simulink model "DIGITAL_TWIN_MPC"  (R2023b)
settings: Solver=FixedStepAuto  StartTime=0.0  StopTime=inf  FixedStep=0.005  RelTol=1e-3  EnableMultiTasking=on
undefined symbols (not defined in the file or in its folder): DiscIntNeverNeededParam, HIL, qc_get_step_size
libraries: quarc_library x6
settings Model: ExtModeTrigDuration=10000  Creator=franc  LastModifiedBy=franc
settings SolverCC: AlgebraicLoopSolver=TrustRegion  PositivePriorityOrder=on
settings DataIOCC: ReturnWorkspaceOutputs=off
settings OptimizationCC: LifeSpan=inf
settings DebuggingCC: UnconnectedInputMsg=warning  UnconnectedOutputMsg=warning  UnconnectedLineMsg=warning  ArithmeticOperatorsInVariantConditions=warning
settings ModelReferenceCC: EnableRefExpFcnMdlSchedulingChecks=on
settings SFSimCC: SimUseLocalCustomCode=off  CustomCodeUndefinedFunction=UseInterfaceOnly
settings RTWCC: Description=QUARC Win64 Target  SystemTargetFile=quarc_win64.tlc  TemplateMakefile=quarc_default_tmf  RTWUseLocalCustomCode=off
settings CodeAppCC: StateflowObjectComments=on
settings STFCustomTargetCC: TargetPreCompLibLocation=C:\PROGRA~3\QUARC\lib\2016a\win64\release  ConcurrentExecutionCompliant=on  GRTInterface=on  SystemTargetFile=quarc_win64.tlc
settings GRTTargetCC: TargetPreCompLibLocation=C:\PROGRA~3\QUARC\lib\2016a\win64\release  ParMdlRefBuildCompliant=off  CompOptLevelCompliant=off  CombineOutputUpdateFcns=off  MatFileLogging=off  CPPClassGenCompliant=off  GRTInterface=on  UseToolchainInfoCompliant=off  ExtMode=on  ExtModeMexFile=quarc_comm
settings ConfigComp: CovMetricSettings=dswe

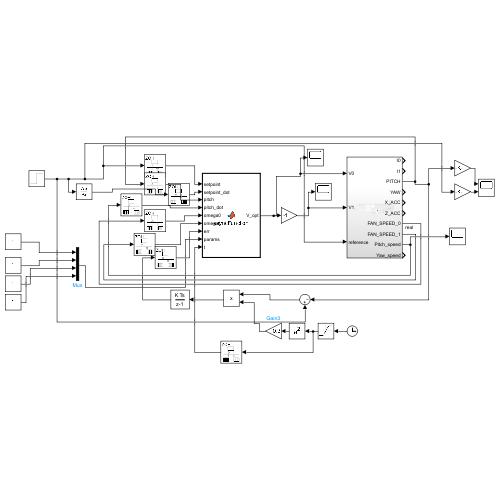
[thumbnail: Simulink's stored preview of the top-level diagram]
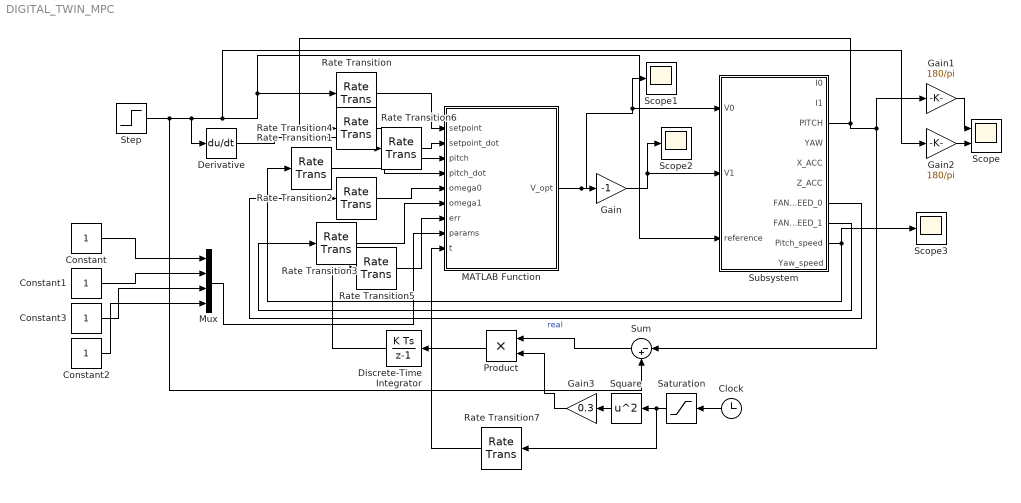
== system DIGITAL_TWIN_MPC ==
  Clock : Clock
  Constant{,1..3} (4 alike) : Constant
  Derivative : Derivative
  Discrete-Time Integrator : DiscreteIntegrator  SampleTime=-1  ICPrevOutput=DiscIntNeverNeededParam  ICPrevScaledInput=DiscIntNeverNeededParam
  Gain : Gain  Gain=-1
  Gain1 : Gain  Gain=180/pi
  Gain2 : Gain  Gain=180/pi
  Gain3 : Gain  Gain=0.3
  MATLAB Function : MATLAB Function  TreatAsAtomicUnit=on  SystemSampleTime=0.1
  Mux : Mux
  Product : Product
  Rate Transition{,1..7} (8 alike) : RateTransition
  Saturation : Saturate  UpperLimit=10  LowerLimit=0
  Scope : Scope  NumInputPorts=2
  Scope1 : Scope
  Scope2 : Scope
  Scope3 : Scope
  Square : Math  Operator=square
  Step : Step  After=30*pi/180  SampleTime=0
  Subsystem : Subsystem
  Sum : Sum  Inputs=|-+
  wires:
  Derivative/1 -> Rate Transition6/1
  Rate Transition4/1 -> MATLAB Function/3(pitch)
  Subsystem/9(Pitch_speed) -> Rate Transition1/1, Scope3/1
  Subsystem/7(FAN_SPEED_0) -> Rate Transition2/1  "real"
  Step/1 -> Sum/2, Derivative/1, Gain2/1, Subsystem/3(reference), Rate Transition/1
  Rate Transition5/1 -> MATLAB Function/7(err)
  Sum/1 -> Product/1
  Discrete-Time Integrator/1 -> Rate Transition5/1
  Gain/1 -> Subsystem/2(V1), Scope2/1
  Rate Transition1/1 -> MATLAB Function/4(pitch_dot)
  Subsystem/8(FAN_SPEED_1) -> Rate Transition3/1
  Rate Transition2/1 -> MATLAB Function/5(omega0)
  MATLAB Function/1(V_opt) -> Gain/1, Scope1/1, Subsystem/1(V0)
  Rate Transition/1 -> MATLAB Function/1(setpoint)
  Rate Transition3/1 -> MATLAB Function/6(omega1)
  Rate Transition6/1 -> MATLAB Function/2(setpoint_dot)
  Subsystem/3(PITCH) -> Gain1/1, Sum/1, Rate Transition4/1
  Gain1/1 -> Scope/1
  Gain2/1 -> Scope/2
  Mux/1 -> MATLAB Function/8(params)
  Rate Transition7/1 -> MATLAB Function/9(t)
  Constant/1 -> Mux/1
  Constant1/1 -> Mux/2
  Constant3/1 -> Mux/3
  Constant2/1 -> Mux/4
  Product/1 -> Discrete-Time Integrator/1
  Saturation/1 -> Rate Transition7/1, Square/1
  Square/1 -> Gain3/1
  Gain3/1 -> Product/2
  Clock/1 -> Saturation/1

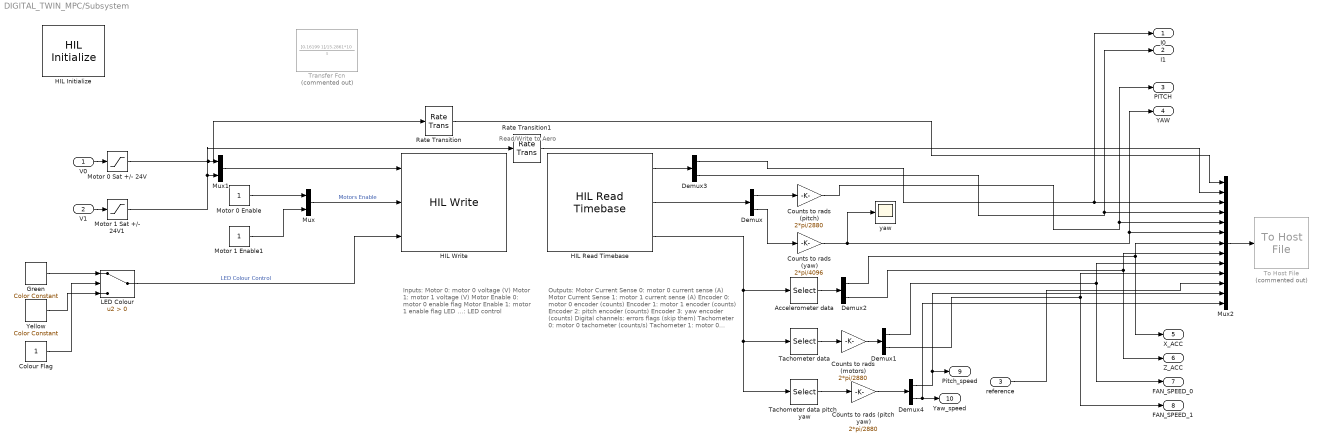
== system DIGITAL_TWIN_MPC/Subsystem ==
  note: Read/Write to Aero
  note: Outputs:
      | Motor Current Sense 0: motor 0 current sense (A)
      | Motor Current Sense 1: motor 1 current sense (A)
      |
      | Encoder 0: motor 0 encoder (counts)
      | Encoder 1: motor 1 encoder (counts)
      | Encoder 2: pitch encoder (counts)
      | Encoder 3: yaw encoder (counts)
      |
      | Digital channels: errors flags (skip them)
      |
      | Tachometer 0: motor 0 tachometer (counts/s)
      | Tachometer 1: motor 0 tachometer (counts/s)
      | Tachometer 2: pitch tachometer (counts/s)
      | Tachometer 3: yaw tachometer (counts/s)
      | Gyro X axis: angular velocity about X axis (rad/s)
      | Gyro Y axis: angular velocity about Y axis (rad/s)
      | Gyro Z axis: angular velocity about Z axis (rad/s)
      | Acceleration X axis: acceleration along X axis (m/s^2)
      | Acceleration Y axis: acceleration along Y axis (m/s^2)
      | Acceleration Z axis: acceleration along Z axis (m/s^2)
  note: Inputs:
      | 	Motor 0: motor 0 voltage (V)
      | 	Motor 1: motor 1 voltage (V)
      |
      | 	Motor Enable 0: motor 0 enable flag
      | 	Motor Enable 1: motor 1 enable flag
      |
      | 	LED ...: LED control
  V0 : Inport
  V1 : Inport  Port=2
  reference : Inport  Port=3
  Accelerometer data : Selector  InputPortWidth=6  IndexOptions=Index vector (dialog)  Indices=[1 2]  OutputSizes=1
  Colour Flag : Constant
  Counts to rads (motors) : Gain  Gain=2*pi/2880
  Counts to rads (pitch yaw) : Gain  Gain=2*pi/2880
  Counts to rads (pitch) : Gain  Gain=2*pi/2880
  Counts to rads (yaw) : Gain  Gain=2*pi/4096
  Demux{,1..4} (5 alike) : Demux  Outputs=2
  Green : quarc_library/Sources/Signals/Color Constant  color=[0 1 0]
      settings: SourceProductName=QUARC Targets
  HIL Initialize : quarc_library/Data Acquisition/Generic/Configuration/HIL Initialize  Priority=-99  object_name=HIL-1  board_type=quanser_aero2_usb  board_number=0@tcpip://localhost:18950  board_options=""  exclusive=off  active=on  hardware_clocks=[0]  clock_modes=[]  initial_clock_frequencies=[]  set_clock_params_at_start=off  set_clock_params_at_switch_in=off  set_clock_frequencies_at_start=off  set_clock_frequencies_at_switch_in=off  analog_input_channels=[0:1]  analog_input_configurations=[]  analog_input_maximums=3  analog_input_minimums=-3  set_analog_input_params_at_start=off  set_analog_input_params_at_switch_in=off  analog_output_channels=[0:1]  analog_output_maximums=24  analog_output_minimums=-24  initial_analog_outputs=[0]  final_analog_outputs=[0]  watchdog_analog_outputs=[0]  set_analog_output_params_at_start=off  set_analog_output_params_at_switch_in=off  set_analog_outputs_at_start=on  set_analog_outputs_at_switch_in=off  set_analog_outputs_at_terminate=on  set_analog_outputs_at_switch_out=off  set_analog_outputs_on_watchdog=on  digital_input_channels=[]  digital_output_channels=[0:1]  digital_output_configuration=[]  initial_digital_outputs=[1]  final_digital_outputs=[0]  watchdog_digital_outputs=[0]  set_digital_output_params_at_start=off  set_digital_output_params_at_switch_in=off  set_digital_outputs_at_start=on  set_digital_outputs_at_switch_in=off  set_digital_outputs_at_terminate=on  set_digital_outputs_at_switch_out=off  set_digital_outputs_on_watchdog=on  encoder_channels=[0:3]  quadrature=[4]  encoder_filter_frequency=[]  initial_encoder_counts=[0]  set_encoder_params_at_start=off  set_encoder_params_at_switch_in=off  set_encoder_counts_at_start=on  set_encoder_counts_at_switch_in=off  pwm_channels=[]  pwm_modes=[]  pwm_frequency=[]  pwm_configuration=[]  pwm_alignment=[]  pwm_polarity=[]  pwm_leading_deadband=[]  pwm_trailing_deadband=[]  initial_pwm_outputs=[]  final_pwm_outputs=[]  watchdog_pwm_outputs=[]  set_pwm_params_at_start=off  set_pwm_params_at_switch_in=off  set_pwm_outputs_at_start=off  set_pwm_outputs_at_switch_in=off  set_pwm_outputs_at_terminate=off  set_pwm_outputs_at_switch_out=off  set_pwm_outputs_on_watchdog=off  other_output_channels=[11000:11002]  initial_other_outputs=[0 1 0]  final_other_outputs=[1 0 0]  watchdog_other_outputs=[0 0 1]  set_other_outputs_at_start=on  set_other_outputs_at_switch_in=off  set_other_outputs_at_terminate=on  set_other_outputs_at_switch_out=off  set_other_outputs_on_watchdog=on
  HIL Read Timebase : quarc_library/Data Acquisition/Generic/Timebases/HIL Read Timebase  object_name=HIL-1  clock=0  analog_channels=[0:1]  encoder_channels=[2:3]  digital_channels=[]  other_channels=[4000 4002 14000:14003 ]  active=on  vector_output=on  data_type_mode=Inherit via back propagation  encoder_data_type=double  digital_data_type=boolean  overflow_mode=Overwrite on overflow  samples_in_buffer=max(ceil(1/qc_get_step_size), 1)
  HIL Write : quarc_library/Data Acquisition/Generic/Immediate I//O/HIL Write  object_name=HIL-1  analog_channels=[0:1]  pwm_channels=[]  digital_channels=[0:1]  other_channels=[11000:11002]  sample_time=-1  active=on  vector_input=on
  LED Colour : Switch  Criteria=u2 > Threshold  SaturateOnIntegerOverflow=off  InputSameDT=off
  Motor 0 Enable : Constant
  Motor 0 Sat +/- 24V : Saturate  UpperLimit=18  LowerLimit=-18
  Motor 1 Enable1 : Constant
  Motor 1 Sat +/- 24V1 : Saturate  UpperLimit=18  LowerLimit=-18
  Mux : Mux  Inputs=2
  Mux1 : Mux  Inputs=2
  Mux2 : Mux  Inputs=13
  Rate Transition : RateTransition
  Rate Transition1 : RateTransition
  Tachometer data : Selector  InputPortWidth=6  IndexOptions=Index vector (dialog)  Indices=[3 4]  OutputSizes=1
  Tachometer data pitch_yaw : Selector  InputPortWidth=6  IndexOptions=Index vector (dialog)  Indices=[5 6]  OutputSizes=1
  To Host File : quarc_library/Sinks/To Host/To Host File  Commented=on  source=Specify via dialog (do not evaluate)  file_name=CONTROLLED_STEP.mat  variable_name=data  decimation=1  sample_time=-1  file_format=MAT-file v.4  options=No header or footer  append=off  final_file_name=CONTROLLED_STEP.mat  bitrate=2000000
  Transfer Fcn : TransferFcn  Commented=on  Numerator=[0.16199 1]/15.2861*10  Denominator=[1 0]
  Yellow : quarc_library/Sources/Signals/Color Constant  color=[1 1 0]
      settings: SourceProductName=QUARC Targets
  yaw : Scope
  I0 : Outport
  I1 : Outport  Port=2
  PITCH : Outport  Port=3
  YAW : Outport  Port=4
  X_ACC : Outport  Port=5
  Z_ACC : Outport  Port=6
  FAN_SPEED_0 : Outport  Port=7
  FAN_SPEED_1 : Outport  Port=8
  Pitch_speed : Outport  Port=9
  Yaw_speed : Outport  Port=10
  wires:
  Demux2/1 -> X_ACC/1, Mux2/7
  Demux2/2 -> Z_ACC/1, Mux2/8
  Demux1/2 -> FAN_SPEED_1/1, Mux2/10
  Demux/1 -> Counts to rads (pitch)/1
  Counts to rads (pitch)/1 -> PITCH/1, Mux2/5
  Motor 0 Sat +/- 24V/1 -> Mux1/1, Rate Transition/1
  Counts to rads (yaw)/1 -> YAW/1, Mux2/6, yaw/1
  Demux1/1 -> FAN_SPEED_0/1, Mux2/9
  Demux3/2 -> I1/1, Mux2/4
  LED Colour/1 -> HIL Write/3  "LED Colour Control"
  V1/1 -> Motor 1 Sat +/- 24V1/1
  HIL Read Timebase/3 -> Tachometer data pitch_yaw/1, Tachometer data/1, Accelerometer data/1
  Mux2/1 -> To Host File/1
  Demux3/1 -> I0/1, Mux2/3
  Counts to rads (motors)/1 -> Demux1/1
  Yellow/1 -> LED Colour/3
  Green/1 -> LED Colour/1
  Mux/1 -> HIL Write/2  "Motors Enable"
  Motor 1 Sat +/- 24V1/1 -> Mux1/2, Rate Transition1/1
  Motor 1 Enable1/1 -> Mux/2
  HIL Read Timebase/2 -> Demux/1
  HIL Read Timebase/1 -> Demux3/1
  Tachometer data/1 -> Counts to rads (motors)/1
  V0/1 -> Motor 0 Sat +/- 24V/1
  Mux1/1 -> HIL Write/1
  Colour Flag/1 -> LED Colour/2
  Demux/2 -> Counts to rads (yaw)/1
  Motor 0 Enable/1 -> Mux/1
  Accelerometer data/1 -> Demux2/1
  reference/1 -> Mux2/11
  Tachometer data pitch_yaw/1 -> Counts to rads (pitch yaw)/1
  Counts to rads (pitch yaw)/1 -> Demux4/1
  Demux4/1 -> Pitch_speed/1, Mux2/12
  Demux4/2 -> Yaw_speed/1, Mux2/13
  Rate Transition/1 -> Mux2/1
  Rate Transition1/1 -> Mux2/2

== matlab function DIGITAL_TWIN_MPC/MATLAB Function ==
  data: setpoint input; setpoint_dot input; V_opt output; pitch input; pitch_dot input; omega0 input; omega1 input; err input; params input; t input
function V_opt = asyncFunction(setpoint,setpoint_dot,pitch,pitch_dot,omega0,omega1,err,params,t)
    fun=@(V)simulate_pitch(0.1,[omega0,omega1,pitch_dot,pitch,err],V,setpoint,setpoint_dot,params,t);
    opts=optimoptions("fmincon","Algorithm","sqp","MaxFunctionEvaluations",1e7);
    size=10;
    V_opt_full=fmincon(fun,ones(size,1),[eye(size);-eye(size)],[18*ones(size,1);18*ones(size,1)],[], [],[],[],[],opts);
    V_opt=V_opt_full(1);
end
